simulink model "AEB_Baseline"  (R2024b)
settings: Solver=VariableStepAuto  StartTime=0.0  StopTime=4  RelTol=1e-3
libraries: simulink x1
settings Model: Creator=garvi  LastModifiedBy=garvi

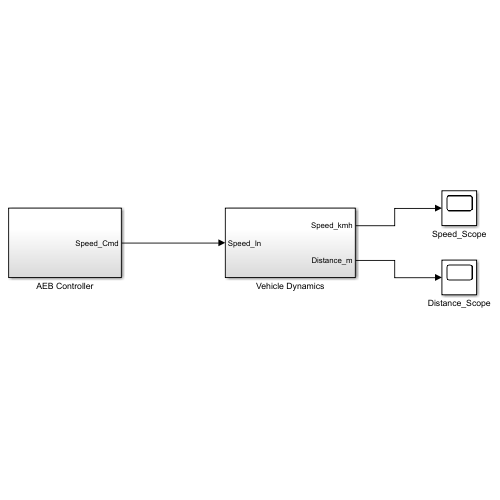
[thumbnail: Simulink's stored preview of the top-level diagram]
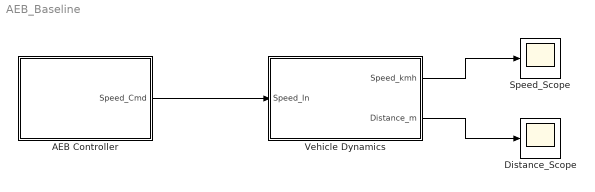
== system AEB_Baseline ==
  AEB Controller : Subsystem
  Distance_Scope : Scope
  Speed_Scope : Scope
  Vehicle Dynamics : Subsystem
  wires:
  AEB Controller/1(Speed_Cmd) -> Vehicle Dynamics/1(Speed_In)
  Vehicle Dynamics/1(Speed_kmh) -> Speed_Scope/1
  Vehicle Dynamics/2(Distance_m) -> Distance_Scope/1

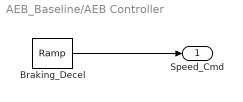
== system AEB_Baseline/AEB Controller ==
  Braking_Decel : simulink/Sources/Ramp  slope=-7.85  start=0  InitialOutput=27.78
  Speed_Cmd : Outport
  wires:
  Braking_Decel/1 -> Speed_Cmd/1

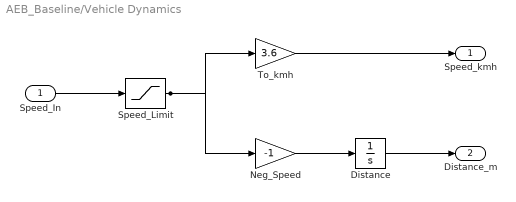
== system AEB_Baseline/Vehicle Dynamics ==
  Speed_In : Inport
  Distance : Integrator  InitialCondition=80  LimitOutput=on  LowerSaturationLimit=0
  Neg_Speed : Gain  Gain=-1
  Speed_Limit : Saturate  UpperLimit=27.78  LowerLimit=0
  To_kmh : Gain  Gain=3.6
  Speed_kmh : Outport
  Distance_m : Outport  Port=2
  wires:
  Speed_In/1 -> Speed_Limit/1
  Speed_Limit/1 -> To_kmh/1, Neg_Speed/1
  Neg_Speed/1 -> Distance/1
  To_kmh/1 -> Speed_kmh/1
  Distance/1 -> Distance_m/1
